simulink model "MPC_quat6DoF"  (R2024b)
settings: Solver=VariableStepAuto  StartTime=0.0  StopTime=5  RelTol=1e-3
model workspace (MAT data in the model file):
  com_error = 0
  controller_type : ControllerType (value not decoded)
  cost_u = [1 0 0]
  cost_x = [0 0 0 0 0 0 0 0 0 0 1]
  discrepancy = 0.5
  dof : object (value not decoded)
  dtime = 0.3
  enable_turbulence = 0
  g = 9.8
  inertia_error = 0
  mass_error = 0
  max_gimbal_rate = 5
  max_iter = 400
  max_throttle_rate = 0.5
  nominal_val = 5
  optimization_time = 0.5
  steps = 50
  stop_time = 100
  u0 = [0 0 0]
  vehicle = Vehicle
  vehicle.m = 100000
  vehicle.L = 30
  vehicle.I = 30000000
  vehicle.Len = 60
  vehicle.max_gimbal = 0.174532925199
  vehicle.min_thrust = 440000
  vehicle.max_thrust = 2210000
  vehicle.Name = "Astra2"
  x0 = [0 100 100 0 0 0 0 -1.57079632679 0 0 0]
  xf = [0 0 0 0 0 0 0 -1.57079632679 0 0 0]
libraries: simulink_extras x2, aerolibanim x1, sharedTrackingLibrary x1, sharedtransform x1, sldrtlib x1, SignalEditorBlockLib x1
settings Model: Creator=alexa  LastModifiedBy=thatf

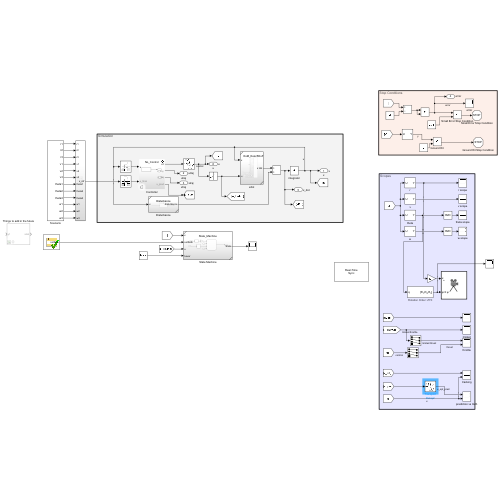
[thumbnail: Simulink's stored preview of the top-level diagram]
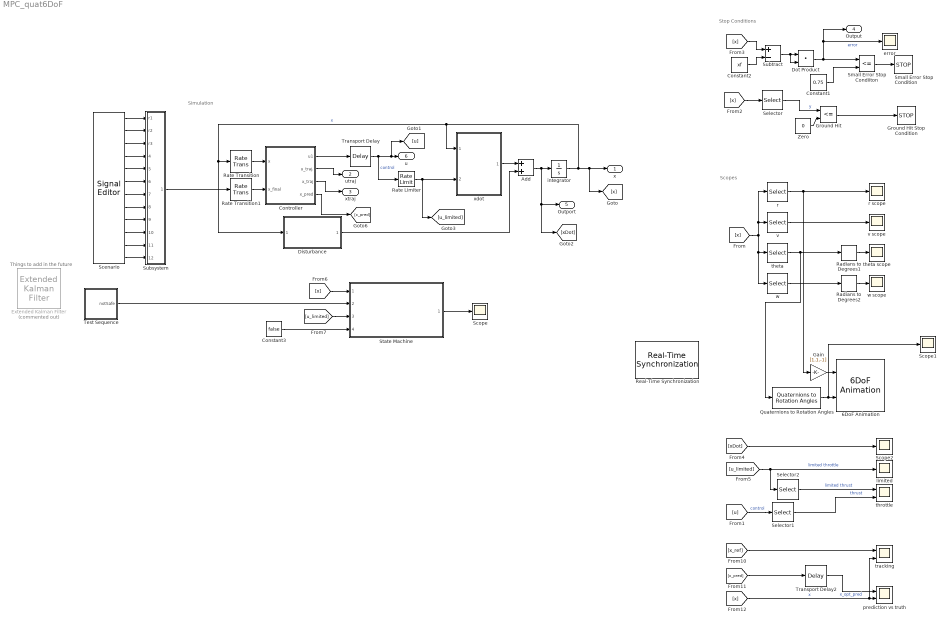
== system MPC_quat6DoF ==
  note: Simulation
  note: Stop Conditions
  note: Things to add in the future
  note: Scopes
  6DoF Animation : aerolibanim/6DoF Animation  u1=[-100 100 -100 100 -800 0]  u2=0.1  u3=10.0  u4=[0, 0, 0]  u5=Fly alongside  u6=[0,80,-50]  u7=40  u8=on
  Add : Sum
  Constant1 : Constant  Value=0.75
  Constant2 : Constant  Value=xf
  Constant3 : Constant  Value=false
  Controller : Subsystem  Variant=on  VariantChoicesSpecifier={}  VariantChoicesEnumeration=ControllerType  VariantControlVariable=controller_type
  Disturbance : Subsystem  ReferencedSubsystem=Disturbance
  Dot Product : DotProduct  OutDataTypeStr=Inherit: Inherit via internal rule
  Extended Kalman Filter : sharedTrackingLibrary/Extended Kalman Filter  Commented=on  StateTransitionFcn=myStateTransitionFcn  HasStateTransitionJacobianFcn=off  HasAdditiveProcessNoise=Additive  ProcessNoise=1  HasTimeVaryingProcessNoise=off  HasStateTransitionFcnExtraArgument=0  InitialState=0  InitialStateCovariance=1  MeasurementFcn1=myMeasurementFcn  HasMeasurementJacobianFcn1=off  HasMeasurementEnablePort1=off  HasAdditiveMeasurementNoise1=Additive  MeasurementNoise1=1  HasTimeVaryingMeasurementNoise1=off  HasMeasurementFcnExtraArgument1=0  HasMeasurementWrapping1=off  MeasurementFcn2=myMeasurementFcn  HasMeasurementJacobianFcn2=off  HasMeasurementEnablePort2=off  HasAdditiveMeasurementNoise2=Additive  MeasurementNoise2=1  HasTimeVaryingMeasurementNoise2=off  HasMeasurementFcnExtraArgument2=0  HasMeasurementWrapping2=off  MeasurementFcn3=myMeasurementFcn  HasMeasurementJacobianFcn3=off  HasMeasurementEnablePort3=off  HasAdditiveMeasurementNoise3=Additive  MeasurementNoise3=1  HasTimeVaryingMeasurementNoise3=off  HasMeasurementFcnExtraArgument3=0  HasMeasurementWrapping3=off  MeasurementFcn4=myMeasurementFcn  HasMeasurementJacobianFcn4=off  HasMeasurementEnablePort4=off  HasAdditiveMeasurementNoise4=Additive  MeasurementNoise4=1  HasTimeVaryingMeasurementNoise4=off  HasMeasurementFcnExtraArgument4=0  HasMeasurementWrapping4=off  MeasurementFcn5=myMeasurementFcn  HasMeasurementJacobianFcn5=off  HasMeasurementEnablePort5=off  HasAdditiveMeasurementNoise5=Additive  MeasurementNoise5=1  HasTimeVaryingMeasurementNoise5=off  HasMeasurementFcnExtraArgument5=0  HasMeasurementWrapping5=off  EnableMultirate=off  StateTransitionFcnSampleTime=1  MeasurementFcn1SampleTime=1  MeasurementFcn2SampleTime=1  MeasurementFcn3SampleTime=1  MeasurementFcn4SampleTime=1  MeasurementFcn5SampleTime=1  UseCurrentEstimator=on  OutputStateCovariance=off  DataType=double  SampleTime=1  NumberOfMeasurements=1
  Gain : Gain  Gain=[1,1,-1]
  Ground Hit : RelationalOperator  Operator=<=  OutDataTypeStr=boolean  RndMeth=Simplest  InputSameDT=off
  Ground Hit Stop Condition : Stop
  Quaternions to Rotation Angles : sharedtransform/Quaternions to Rotation Angles  rotationOrder=ZYX  aMode=aMode
  Radians to Degrees1 : simulink_extras/Transformations/Radians to Degrees
  Radians to Degrees2 : simulink_extras/Transformations/Radians to Degrees
  Rate Limiter : RateLimiter  RisingSlewLimit=max_throttle_rate*100  FallingSlewLimit=-max_throttle_rate *100  SampleTimeMode=inherited  InitialCondition=u0
  Rate Transition : RateTransition  InitialCondition=x0  OutPortSampleTime=optimization_time
  Rate Transition1 : RateTransition  InitialCondition=xf  OutPortSampleTime=optimization_time
  Real-Time Synchronization : sldrtlib/Real-Time Synchronization  SampleTime=0.1  MaxMissedTicks=10  ShowMissedTicks=off  YieldWhenWaiting=off
  Scenario : SignalEditorBlockLib/Signal Editor  FileName=land_at_origin_scenario.mat  ActiveScenario=Scenario  ActiveSignal=r1  IsBus=off  OutputBusObjectStr=Bus: BusObject  SampleTime=0  ZeroCross=off  OutputAfterFinalValue=Holding final value  Unit=inherit  PreserveSignalName=on  ApplySigPropsToAllScenarios=on  ApplySigPropsToAllSignals=on
  Scope : Scope
  Scope1 : Scope
  Scope2 : Scope
  Selector : Selector  InputPortWidth=dof.nx  IndexOptions=Index vector (dialog)  Indices=[2]  OutputSizes=1
  Selector1 : Selector  InputPortWidth=dof.nu  IndexOptions=Index vector (dialog)  Indices=dof.ithrust  OutputSizes=1
  Selector2 : Selector  InputPortWidth=dof.nu  IndexOptions=Index vector (dialog)  Indices=dof.ithrust  OutputSizes=1
  Small Error Stop Condiiton : RelationalOperator  Operator=<=  OutDataTypeStr=boolean  RndMeth=Simplest  InputSameDT=off
  Small Error Stop Condition : Stop
  State Machine : Subsystem  ReferencedSubsystem=State_Machine
  Subsystem : Subsystem
  Subtract : Sum  Inputs=+-
  Test Sequence : Test Sequence  TreatAsAtomicUnit=on
  Transport Delay : TransportDelay  DelayTime=optimization_time  InitialOutput=u0 + [0.4,0,0]
  Transport Delay2 : TransportDelay  DelayTime=optimization_time  InitialOutput=x0'
  Zero : Constant  Value=0  OutDataTypeStr=Inherit: Inherit via back propagation
  error : Scope
  integrator : Integrator  InitialCondition=x0
  limited : Scope
  prediction vs truth : Scope  NumInputPorts=2
  r : Selector  InputPortWidth=dof.nx  IndexOptions=Index vector (dialog)  Indices=dof.ir  OutputSizes=1
  r scope : Scope
  theta : Selector  InputPortWidth=dof.nx  IndexOptions=Index vector (dialog)  Indices=dof.itheta  OutputSizes=1
  theta scope : Scope
  throttle : Scope  NumInputPorts=2
  tracking : Scope  NumInputPorts=2
  v : Selector  InputPortWidth=dof.nx  IndexOptions=Index vector (dialog)  Indices=dof.iv  OutputSizes=1
  v scope : Scope
  w : Selector  InputPortWidth=dof.nx  IndexOptions=Index vector (dialog)  Indices=dof.iw  OutputSizes=1
  w scope : Scope
  xdot : Subsystem  ReferencedSubsystem=EoM_Euler5DoF
  x : Outport  SignalName=x
  utraj : Outport  Port=2  SignalName=utraj
  xtraj : Outport  Port=3  SignalName=xtraj
  Output : Outport  Port=4  SignalName=error
  Outport : Outport  Port=5  SignalName=x_dot
  u : Outport  Port=6  SignalName=u
  wires:
  xdot/1 -> Add/1
  integrator/1 -> Disturbance/1, Rate Transition/1, xdot/1, x/1, [x]  "x"
  Controller/3(x_traj) -> xtraj/1
  Transport Delay/1 -> [u], u/1, Rate Limiter/1  "control"
  Controller/2(u_traj.) -> utraj/1
  Add/1 -> integrator/1, [xDot], Outport/1
  Rate Transition/1 -> Controller/1(x)
  Disturbance/1 -> Add/2
  Controller/1(u1) -> Transport Delay/1
  Ground Hit/1 -> Ground Hit Stop Condition/1
  Constant1/1 -> Small Error Stop Condiiton/2
  Constant2/1 -> Subtract/2
  Selector/1 -> Ground Hit/1  "y"
  Dot Product/1 -> Output/1, error/1, Small Error Stop Condiiton/1  "error"
  Subtract/1 -> Dot Product/2, Dot Product/1
  [x] -> Selector/1
  Zero/1 -> Ground Hit/2
  [x] -> Subtract/1
  Small Error Stop Condiiton/1 -> Small Error Stop Condition/1
  Rate Limiter/1 -> [u_limited], xdot/2
  Rate Transition1/1 -> Controller/2(x_final)
  Controller/4(x_pred) -> [x_pred]
  Test Sequence/1(notSafe) -> State Machine/2
  [x] -> State Machine/1
  [u_limited] -> State Machine/3
  Constant3/1 -> State Machine/4
  State Machine/1 -> Scope/1
  [x_ref] -> tracking/1
  Transport Delay2/1 -> prediction vs truth/1  "x_opt_pred"
  [u] -> Selector1/1  "control"
  [x] -> tracking/2, prediction vs truth/2  "x"
  [u_limited] -> Selector2/1, limited/1  "limited throttle"
  [x_pred] -> Transport Delay2/1
  [xDot] -> Scope2/1
  Scenario/1 -> Subsystem/1(r1)
  Scenario/2 -> Subsystem/2(r2)
  Scenario/3 -> Subsystem/3(r3)
  Scenario/4 -> Subsystem/4(v1)
  Scenario/5 -> Subsystem/5(v2)
  Scenario/6 -> Subsystem/6(v3)
  Scenario/7 -> Subsystem/7(theta1)
  Scenario/8 -> Subsystem/8(theta2)
  Scenario/9 -> Subsystem/9(theta3)
  Scenario/10 -> Subsystem/10(w1)
  Scenario/11 -> Subsystem/11(w2)
  Scenario/12 -> Subsystem/12(w3)
  Subsystem/1(x_ref) -> Rate Transition1/1
  [x] -> w/1, theta/1, v/1, r/1
  w/1 -> Radians to Degrees2/1
  r/1 -> Gain/1, r scope/1
  v/1 -> v scope/1
  Quaternions to Rotation Angles/1 -> Scope1/1, 6DoF Animation/2
  Gain/1 -> 6DoF Animation/1
  Radians to Degrees1/1 -> theta scope/1
  Radians to Degrees2/1 -> w scope/1
  theta/1 -> Quaternions to Rotation Angles/1, Radians to Degrees1/1
  Selector1/1 -> throttle/2  "thrust"
  Selector2/1 -> throttle/1  "limited thrust"

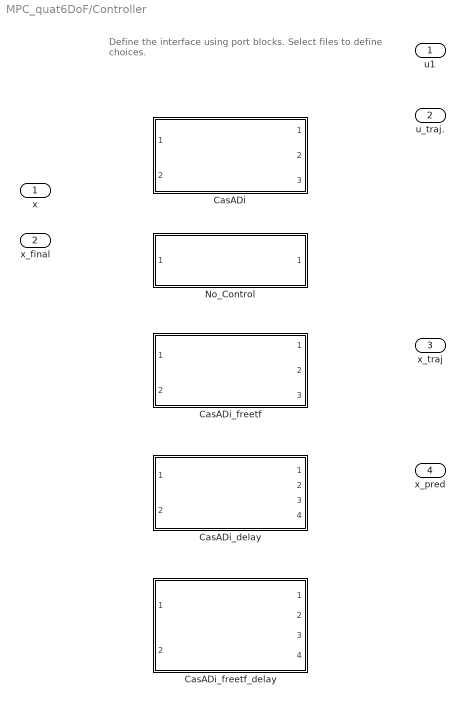
== system MPC_quat6DoF/Controller ==
  note: Define the interface using port blocks.
      | Select files to define choices.
  x : Inport
  x_final : Inport  Port=2
  CasADi : Subsystem  VariantControl=controller_type == ControllerType.CasADi  ReferencedSubsystem=CasADi
  CasADi_delay : Subsystem  VariantControl=controller_type == ControllerType.CasADi_delay  ReferencedSubsystem=CasADi_delay
  CasADi_freetf : Subsystem  VariantControl=controller_type == ControllerType.CasADi_freetf  ReferencedSubsystem=CasADi_freetf
  CasADi_freetf_delay : Subsystem  VariantControl=controller_type == ControllerType.CasADi_freetf_delay  ReferencedSubsystem=CasADi_freetf_delay
  No_Control : Subsystem  VariantControl=controller_type == ControllerType.No_Control  ReferencedSubsystem=No_Control
  u1 : Outport
  u_traj. : Outport  Port=2
  x_traj : Outport  Port=3
  x_pred : Outport  Port=4

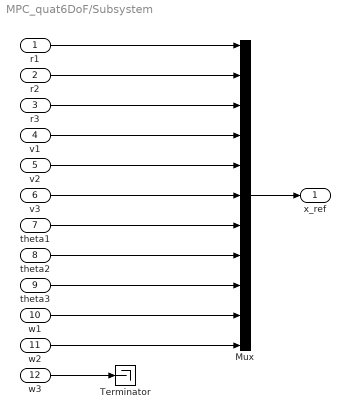
== system MPC_quat6DoF/Subsystem ==
  r1 : Inport
  r2 : Inport  Port=2
  r3 : Inport  Port=3
  v1 : Inport  Port=4
  v2 : Inport  Port=5
  v3 : Inport  Port=6
  theta1 : Inport  Port=7
  theta2 : Inport  Port=8
  theta3 : Inport  Port=9
  w1 : Inport  Port=10
  w2 : Inport  Port=11
  w3 : Inport  Port=12
  Mux : Mux  Inputs=11
  Terminator : Terminator
  x_ref : Outport
  wires:
  Mux/1 -> x_ref/1
  r1/1 -> Mux/1
  r2/1 -> Mux/2
  r3/1 -> Mux/3
  v1/1 -> Mux/4
  v2/1 -> Mux/5
  v3/1 -> Mux/6
  theta1/1 -> Mux/7
  theta2/1 -> Mux/8
  theta3/1 -> Mux/9
  w1/1 -> Mux/10
  w2/1 -> Mux/11
  w3/1 -> Terminator/1

== stateflow chart MPC_quat6DoF/Test Sequence ==
  state Scenario_1
    state step_1
    state step_2
      notSafe = true;
    (default) -> step_1
    step_1 -> step_2 : [
        | after(5, sec)
        | ]
  (default) -> Scenario_1 : {assert(Active_Scenario_Index == 1,'The value of Scenario Parameter ''Active_Scenario_Index'' is not valid. Use the index of the scenario to specify it.')}
  data: Active_Scenario_Index parameter =1; notSafe output
